simulink model "SIM002"  (R2019a)
settings: Solver=FixedStepAuto  StartTime=0.0  StopTime=20  FixedStep=0.0001  RelTol=1e-3
values from neighbouring files (symbols this model uses):
  A = 4    [SIM002.m]    (also in SIM004_DIMENSIONAL_PARAMS.m = 12)
  c = c_st + c_gen    (= 0.1024)    [SIM001.m]    (also in SIM004_DIMENSIONAL_PARAMS.m = 0)
  c2 = rho_w*Cd*D*L/2    (= 12.8)    [SIM001.m]
  F0 = rho_w*D*U^2*L*sqrt(2)*CL_rms/2    [SIM001.m]
  fv = St*U/D    [SIM001.m]
  k = 200    [SIM001.m]    (also in SIM002.m = 280; SIM004_DIMENSIONAL_PARAMS.m)
  kt = 0.032    [SIM001.m]    (also in SIM004_DIMENSIONAL_PARAMS.m = 0.1)
  M = m + m_h    (= 4.82548631591)    [SIM001.m]    (also in SIM002.m = 5.6587609211; SIM004_DIMENSIONAL_PARAMS.m = 5.6587609211)
  r2 = 0.01    [SIM001.m]    (also in SIM004_DIMENSIONAL_PARAMS.m)
libraries: powerlib x5, powerlib_meascontrol x1
settings Model: Creator=dinet  LastModifiedBy=dinet

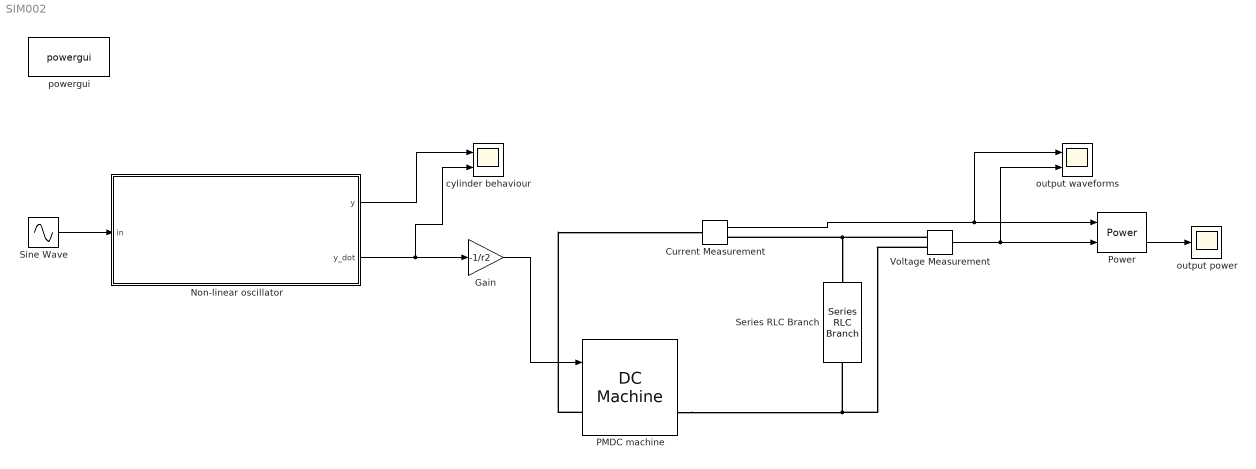
== system SIM002 ==
  Current Measurement : powerlib/Measurements/Current Measurement  PhasorSimulation=off  OutputType=Complex  PSBequivalent=0
      settings: SourceProductName=Simscape Electrical
  Gain : Gain  Gain=-1/r2
  Non-linear oscillator : Subsystem
  "PMDC machine " : powerlib/Machines/DC Machine  PresetModel=No  MechanicalLoad=Speed w  FieldType=Permanent magnet  ShowDetailedParameters=on  MeasurementBus=off  RLa="[ 0.6  0.012]"  RLf="[ 240  120]"  Laf=1.8  MachineConstant=Torque constant (N.m/A)  Ke=0.003  Kt=kt  J=1  Bm=0  Tf=0  w0=1  Ifinit=1  TsPowergui=0  TsBlock=-1
      settings: SourceProductName=Simscape Electrical
  Power : powerlib_meascontrol/Measurements/Power  Freq=fv  Vinit=[0, 0]  Iinit=[0, 0]  Ts=0
      settings: SourceProductName=Simscape Electrical
  Series RLC Branch : powerlib/Elements/Series RLC Branch  LConnTagsString=__new0  RConnTagsString=__new0  BranchType=R  Resistance=100  Inductance=0  SetiL0=off  InitialCurrent=0  Capacitance=0  Setx0=off  InitialVoltage=0  Measurements=None
      settings: SourceProductName=Simscape Electrical
  Sine Wave : Sin  Frequency=2*pi*fv  SampleTime=0
  Voltage Measurement : powerlib/Measurements/Voltage Measurement  PhasorSimulation=off  OutputType=Complex  PSBequivalent=0
      settings: SourceProductName=Simscape Electrical
  cylinder behaviour : Scope  NumInputPorts=2
  output power : Scope
  output waveforms : Scope  NumInputPorts=2
  powergui : powerlib/powergui  Priority=1  SimulationMode=Continuous  SampleTime=50e-6  frequency=60  Iterations=50  frequencyindice=0  Pbase=100e6  ErrMax=1e-4  UnitsV=kV  UnitsW=MW  buscounter=0  FunctionMessages=off  echomessages=off  EnableUseOfTLC=off  CurrentSourceSwitches=off  DisableSnubberDevices=off  DisableRonSwitches=off  DisableVfSwitches=off  DisplayEquations=off  AutomaticDiscreteSolvers=off  SolverType=Tustin/Backward Euler (TBE)  Interpol=off  ExternalGateDelay=off  methode=off  Ts=100  x0status=blocks  SPID=on  SwTol=0  HookPort=off  NonlinearTolerance=0  nMaxIteration=15  ContinueOnMaxIteration=off  RestoreLinks=warning  ResistiveCurrentMeasurement=off  Frange=[0:2:500]  Ylog=off  Xlog=on  ShowGrid=off  save=off  variable=ZData  structure=0  ZoomFFT=off  StartTime=0.0  cycles=1  DisplayStyle=1  fundamental=60  FreqAxis=off  MaxFrequency=1000  frequencyindicesteady=1  RmsSteady=1  display=off
      settings: SourceProductName=Simscape Electrical
  wires:
  Sine Wave/1 -> Non-linear oscillator/1(in)
  Non-linear oscillator/2(y_dot) -> cylinder behaviour/2, Gain/1
  Gain/1 -> "PMDC machine "/1
  Current Measurement/1 -> output waveforms/1, Power/2
  Voltage Measurement/1 -> output waveforms/2, Power/1
  Power/1 -> output power/1
  Non-linear oscillator/1(y) -> cylinder behaviour/1
  connections:
  Voltage Measurement/LConn1 -- Current Measurement/RConn1 -- Series RLC Branch/LConn1
  Voltage Measurement/LConn2 -- "PMDC machine "/RConn1 -- Series RLC Branch/RConn1
  "PMDC machine "/LConn1 -- Current Measurement/LConn1

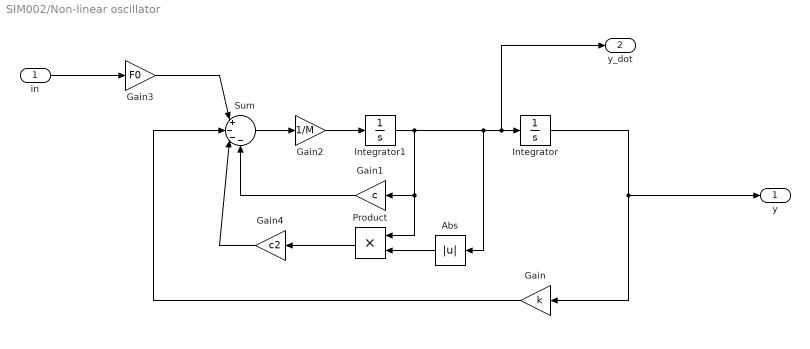
== system SIM002/Non-linear oscillator ==
  in : Inport
  Abs : Abs
  Gain : Gain  Gain=k
  Gain1 : Gain  Gain=c
  Gain2 : Gain  Gain=1/M
  Gain3 : Gain  Gain=F0
  Gain4 : Gain  Gain=c2
  Integrator : Integrator
  Integrator1 : Integrator
  Product : Product
  Sum : Sum  Inputs=|+---
  y : Outport
  y_dot : Outport  Port=2
  wires:
  Gain1/1 -> Sum/4
  Gain4/1 -> Sum/3
  Gain2/1 -> Integrator1/1
  Gain/1 -> Sum/2
  Integrator1/1 -> Abs/1, y_dot/1, Integrator/1, Product/1, Gain1/1
  Abs/1 -> Product/2
  Product/1 -> Gain4/1
  Integrator/1 -> y/1, Gain/1
  Gain3/1 -> Sum/1
  Sum/1 -> Gain2/1
  in/1 -> Gain3/1
